simulink model "ddc_eng"  (R2012b)
(part 2 of 50)

      | pipeline_init(gcb,'latency',latency);
      settings: AttributesFormatString=Latency = %<latency>
      mask Display:
      | port_label('input', 1, 'd');
      | port_label('output', 1, 'q');
      | disp(['Z^-', num2str(latency)]);
  pipeline48 : Subsystem  AncestorBlock=casper_library_delays/pipeline  mask(pipeline){latency=2}
      mask help:
      | An explicitly laid-out delay line to avoid mapping to SRL16s
      | for use in pipelining to help achieve timing closure.
      mask init:
      | pipeline_init(gcb,'latency',latency);
      settings: AttributesFormatString=Latency = %<latency>
      mask Display:
      | port_label('input', 1, 'd');
      | port_label('output', 1, 'q');
      | disp(['Z^-', num2str(latency)]);
  pipeline49 : Subsystem  AncestorBlock=casper_library_delays/pipeline  mask(pipeline){latency=2}
      mask help:
      | An explicitly laid-out delay line to avoid mapping to SRL16s
      | for use in pipelining to help achieve timing closure.
      mask init:
      | pipeline_init(gcb,'latency',latency);
      settings: AttributesFormatString=Latency = %<latency>
      mask Display:
      | port_label('input', 1, 'd');
      | port_label('output', 1, 'q');
      | disp(['Z^-', num2str(latency)]);
  pipeline5 : Subsystem  AncestorBlock=casper_library_delays/pipeline  mask(pipeline){latency=2}
      mask help:
      | An explicitly laid-out delay line to avoid mapping to SRL16s
      | for use in pipelining to help achieve timing closure.
      mask init:
      | pipeline_init(gcb,'latency',latency);
      settings: AttributesFormatString=Latency = %<latency>
      mask Display:
      | port_label('input', 1, 'd');
      | port_label('output', 1, 'q');
      | disp(['Z^-', num2str(latency)]);
  pipeline53 : Subsystem  AncestorBlock=casper_library_delays/pipeline  mask(pipeline){latency=2}
      mask help:
      | An explicitly laid-out delay line to avoid mapping to SRL16s
      | for use in pipelining to help achieve timing closure.
      mask init:
      | pipeline_init(gcb,'latency',latency);
      settings: AttributesFormatString=Latency = %<latency>
      mask Display:
      | port_label('input', 1, 'd');
      | port_label('output', 1, 'q');
      | disp(['Z^-', num2str(latency)]);
  pipeline54 : Subsystem  AncestorBlock=casper_library_delays/pipeline  mask(pipeline){latency=2}
      mask help:
      | An explicitly laid-out delay line to avoid mapping to SRL16s
      | for use in pipelining to help achieve timing closure.
      mask init:
      | pipeline_init(gcb,'latency',latency);
      settings: AttributesFormatString=Latency = %<latency>
      mask Display:
      | port_label('input', 1, 'd');
      | port_label('output', 1, 'q');
      | disp(['Z^-', num2str(latency)]);
  pipeline55 : Subsystem  AncestorBlock=casper_library_delays/pipeline  mask(pipeline){latency=2}
      mask help:
      | An explicitly laid-out delay line to avoid mapping to SRL16s
      | for use in pipelining to help achieve timing closure.
      mask init:
      | pipeline_init(gcb,'latency',latency);
      settings: AttributesFormatString=Latency = %<latency>
      mask Display:
      | port_label('input', 1, 'd');
      | port_label('output', 1, 'q');
      | disp(['Z^-', num2str(latency)]);
  pipeline6 : Subsystem  AncestorBlock=casper_library_delays/pipeline  mask(pipeline){latency=2}
      mask help:
      | An explicitly laid-out delay line to avoid mapping to SRL16s
      | for use in pipelining to help achieve timing closure.
      mask init:
      | pipeline_init(gcb,'latency',latency);
      settings: AttributesFormatString=Latency = %<latency>
      mask Display:
      | port_label('input', 1, 'd');
      | port_label('output', 1, 'q');
      | disp(['Z^-', num2str(latency)]);
  pipeline61 : Subsystem  AncestorBlock=casper_library_delays/pipeline  mask(pipeline){latency=2}
      mask help:
      | An explicitly laid-out delay line to avoid mapping to SRL16s
      | for use in pipelining to help achieve timing closure.
      mask init:
      | pipeline_init(gcb,'latency',latency);
      settings: AttributesFormatString=Latency = %<latency>
      mask Display:
      | port_label('input', 1, 'd');
      | port_label('output', 1, 'q');
      | disp(['Z^-', num2str(latency)]);
  pipeline7 : Subsystem  AncestorBlock=casper_library_delays/pipeline  mask(pipeline){latency=2}
      mask help:
      | An explicitly laid-out delay line to avoid mapping to SRL16s
      | for use in pipelining to help achieve timing closure.
      mask init:
      | pipeline_init(gcb,'latency',latency);
      settings: AttributesFormatString=Latency = %<latency>
      mask Display:
      | port_label('input', 1, 'd');
      | port_label('output', 1, 'q');
      | disp(['Z^-', num2str(latency)]);
  pipeline8 : Subsystem  AncestorBlock=casper_library_delays/pipeline  mask(pipeline){latency=2}
      mask help:
      | An explicitly laid-out delay line to avoid mapping to SRL16s
      | for use in pipelining to help achieve timing closure.
      mask init:
      | pipeline_init(gcb,'latency',latency);
      settings: AttributesFormatString=Latency = %<latency>
      mask Display:
      | port_label('input', 1, 'd');
      | port_label('output', 1, 'q');
      | disp(['Z^-', num2str(latency)]);
  pipeline9 : Subsystem  AncestorBlock=casper_library_delays/pipeline  mask(pipeline){latency=2}
      mask help:
      | An explicitly laid-out delay line to avoid mapping to SRL16s
      | for use in pipelining to help achieve timing closure.
      mask init:
      | pipeline_init(gcb,'latency',latency);
      settings: AttributesFormatString=Latency = %<latency>
      mask Display:
      | port_label('input', 1, 'd');
      | port_label('output', 1, 'q');
      | disp(['Z^-', num2str(latency)]);
  pipeline93 : Subsystem  AncestorBlock=casper_library_delays/pipeline  mask(pipeline){latency=2}
      mask help:
      | An explicitly laid-out delay line to avoid mapping to SRL16s
      | for use in pipelining to help achieve timing closure.
      mask init:
      | pipeline_init(gcb,'latency',latency);
      settings: AttributesFormatString=Latency = %<latency>
      mask Display:
      | port_label('input', 1, 'd');
      | port_label('output', 1, 'q');
      | disp(['Z^-', num2str(latency)]);
  pipeline98 : Subsystem  AncestorBlock=casper_library_delays/pipeline  mask(pipeline){latency=2}
      mask help:
      | An explicitly laid-out delay line to avoid mapping to SRL16s
      | for use in pipelining to help achieve timing closure.
      mask init:
      | pipeline_init(gcb,'latency',latency);
      settings: AttributesFormatString=Latency = %<latency>
      mask Display:
      | port_label('input', 1, 'd');
      | port_label('output', 1, 'q');
      | disp(['Z^-', num2str(latency)]);
  pipeline99 : Subsystem  AncestorBlock=casper_library_delays/pipeline  mask(pipeline){latency=2}
      mask help:
      | An explicitly laid-out delay line to avoid mapping to SRL16s
      | for use in pipelining to help achieve timing closure.
      mask init:
      | pipeline_init(gcb,'latency',latency);
      settings: AttributesFormatString=Latency = %<latency>
      mask Display:
      | port_label('input', 1, 'd');
      | port_label('output', 1, 'q');
      | disp(['Z^-', num2str(latency)]);
  receptor_id : Subsystem  Tag=xps:sw_reg  AncestorBlock=xps_library/software register  mask(swreg){mode=fields of arbitrary size, io_dir=From Processor, io_delay=1, sample_period=1, names=[receptor_id pol0_id pol1_id], bitwidths=[14 2 2], arith_types=[0 0 0], bin_pts=[0 0 0], show_format=on}
      mask prompts: io_dir "I/O direction"; io_delay "I/O delay"; sample_period "Sample period"; names "Names [msb ... lsb]:"; bitwidths "Bitwidths [msb ... lsb]:"; arith_types "Types (ufix=0, fix=1, bool=2) [msb ... lsb]:"; bin_pts "Binary pts [msb ... lsb]:"; show_format "Print format string?"
      mask init:
      | swreg_init(gcb)
      settings: AttributesFormatString=3 inputs:uf14.0,uf2.0,uf2.0,
      mask TypeOptions mode: one value | fields of equal size | fields of arbitrary size
      mask Callback mode: swreg_cb(gcb);
      mask TypeOptions io_dir: To Processor | From Processor
      mask Callback io_dir:
      | mask_enables = get_param(gcb, 'MaskEnables');
      | mask_names = get_param(gcb, 'MaskNames');
      | if strcmp(get_param(gcb, 'io_dir'), 'To Processor'),
      |     mask_enables{ismember(mask_names, 'sample_period')} = 'off';
      | else
      |     mask_enables{ismember(mask_names, 'sample_period')} = 'on';
      | end
      | set_param(gcb, 'MaskEnables', mask_enables);
      mask Callback bitwidths:
      | blk = gcb;
      | mode = get_param(blk, 'mode');
      | current_widths = eval(get_param(blk, 'bitwidths'));
      | if (strcmp(mode, 'one value') || strcmp(mode, 'fields of equal size')) && (length(current_widths) > 1),
      |     error('Only one width may be specified for this mode.');
      | elseif strcmp(mode, 'fields of arbitrary size')
      |     current_names = textscan(strtrim(strrep(strrep(get_param(blk, 'names'), ']', ''), '[', '')), '%s');
      |     current_names = current_names{1};
      |     numios = length(current_names);
      |     if length(current_widths) ~= numios,
      |         error('%d field names specified, but %d widths?', numios, length(current_widths));
      |     end
      | end
      | total_width = 0;
      | for ctr = 1 : length(current_widths),
      |     total_width = total_width + current_widths(ctr);
      | end
      | if total_width > 32,
      |     error('Total width must be 32 or less, set to %d.', total_width);
      | end
      mask Callback arith_types:
      | blk = gcb;
      | mode = get_param(blk, 'mode');
      | current_types = eval(get_param(blk, 'arith_types'));
      | numios = length(current_types);
      | if (strcmp(mode, 'one value') || strcmp(mode, 'fields of equal size')) && (length(current_types) > 1),
      |     error('Only one type may be specified for this mode.');
      | elseif strcmp(mode, 'fields of arbitrary size')
      |     current_names = textscan(strtrim(strrep(strrep(get_param(blk, 'names'), ']', ''), '[', '')), '%s');
      |     current_names = current_names{1};
      |     numios = length(current_names);
      |     if length(current_types) ~= numios,
      |         error('%d field names specified, but %d types?', numios, length(current_types));
      |     end
      | end
      | problem = 0;
      | for ctr = 1 : numios,
      |     t = current_types(ctr);
      |     if (t < 0) || (t > 2),
      |         problem = t;
      |         ctr = numios + 1;
      |     end
      | end
      | if problem ~= 0,
      |     error('Type cannot be %i, must be 0, 1 or 2.', problem);
      | end
      mask Callback bin_pts:
      | blk = gcb;
      | mode = get_param(blk, 'mode');
      | current_bins = eval(get_param(blk, 'bin_pts'));
      | if (strcmp(mode, 'one value') || strcmp(mode, 'fields of equal size')) && (length(current_bins) > 1),
      |     error('Only one binary pt may be specified for this mode.');
      | elseif strcmp(mode, 'fields of arbitrary size')
      |     current_names = textscan(strtrim(strrep(strrep(get_param(blk, 'names'), ']', ''), '[', '')), '%s');
      |     current_names = current_names{1};
      |     numios = length(current_names);
      |     if length(current_bins) ~= numios,
      |         error('%d field names specified, but %d binary pts?', numios, length(current_bins));
      |     end
      | end
  reorder_ctrs : Subsystem  Tag=xps:sw_reg  AncestorBlock=xps_library/software register  mask(swreg){mode=fields of arbitrary size, io_dir=To Processor, io_delay=0, sample_period=1, names=[pktof0 pktof1 pktof2 pktof3], bitwidths=[8 8 8 8], arith_types=[0 0 0 0], bin_pts=[0 0 0 0], sim_port=off, show_format=on}
      mask prompts: io_dir "I/O direction"; io_delay "I/O delay"; sample_period "Sample period"; names "Names [msb ... lsb]:"; bitwidths "Bitwidths [msb ... lsb]:"; arith_types "Types (ufix=0, fix=1, bool=2) [msb ... lsb]:"; bin_pts "Binary pts [msb ... lsb]:"; sim_port "Provide sim input/output?"; show_format "Print format string?"
      mask init:
      | swreg_init(gcb)
      settings: AttributesFormatString=4 outputs:uf8.0,uf8.0,uf8.0,uf8.0,
      mask TypeOptions mode: one value | fields of equal size | fields of arbitrary size
      mask Callback mode: swreg_cb(gcb);
      mask TypeOptions io_dir: To Processor | From Processor
      mask Callback io_dir:
      | mask_enables = get_param(gcb, 'MaskEnables');
      | mask_names = get_param(gcb, 'MaskNames');
      | if strcmp(get_param(gcb, 'io_dir'), 'To Processor'),
      |     mask_enables{ismember(mask_names, 'sample_period')} = 'off';
      | else
      |     mask_enables{ismember(mask_names, 'sample_period')} = 'on';
      | end
      | set_param(gcb, 'MaskEnables', mask_enables);
      mask Callback bitwidths:
      | blk = gcb;
      | mode = get_param(blk, 'mode');
      | current_widths = eval(get_param(blk, 'bitwidths'));
      | if (strcmp(mode, 'one value') || strcmp(mode, 'fields of equal size')) && (length(current_widths) > 1),
      |     error('Only one width may be specified for this mode.');
      | elseif strcmp(mode, 'fields of arbitrary size')
      |     current_names = textscan(strtrim(strrep(strrep(get_param(blk, 'names'), ']', ''), '[', '')), '%s');
      |     current_names = current_names{1};
      |     numios = length(current_names);
      |     if length(current_widths) ~= numios,
      |         error('%d field names specified, but %d widths?', numios, length(current_widths));
      |     end
      | end
      | total_width = 0;
      | for ctr = 1 : length(current_widths),
      |     total_width = total_width + current_widths(ctr);
      | end
      | if total_width > 32,
      |     error('Total width must be 32 or less, set to %d.', total_width);
      | end
      mask Callback arith_types:
      | blk = gcb;
      | mode = get_param(blk, 'mode');
      | current_types = eval(get_param(blk, 'arith_types'));
      | numios = length(current_types);
      | if (strcmp(mode, 'one value') || strcmp(mode, 'fields of equal size')) && (length(current_types) > 1),
      |     error('Only one type may be specified for this mode.');
      | elseif strcmp(mode, 'fields of arbitrary size')
      |     current_names = textscan(strtrim(strrep(strrep(get_param(blk, 'names'), ']', ''), '[', '')), '%s');
      |     current_names = current_names{1};
      |     numios = length(current_names);
      |     if length(current_types) ~= numios,
      |         error('%d field names specified, but %d types?', numios, length(current_types));
      |     end
      | end
      | problem = 0;
      | for ctr = 1 : numios,
      |     t = current_types(ctr);
      |     if (t < 0) || (t > 2),
      |         problem = t;
      |         ctr = numios + 1;
      |     end
      | end
      | if problem ~= 0,
      |     error('Type cannot be %i, must be 0, 1 or 2.', problem);
      | end
      mask Callback bin_pts:
      | blk = gcb;
      | mode = get_param(blk, 'mode');
      | current_bins = eval(get_param(blk, 'bin_pts'));
      | if (strcmp(mode, 'one value') || strcmp(mode, 'fields of equal size')) && (length(current_bins) > 1),
      |     error('Only one binary pt may be specified for this mode.');
      | elseif strcmp(mode, 'fields of arbitrary size')
      |     current_names = textscan(strtrim(strrep(strrep(get_param(blk, 'names'), ']', ''), '[', '')), '%s');
      |     current_names = current_names{1};
      |     numios = length(current_names);
      |     if length(current_bins) ~= numios,
      |         error('%d field names specified, but %d binary pts?', numios, length(current_bins));
      |     end
      | end
  reorder_ctrs1 : Subsystem  Tag=xps:sw_reg  AncestorBlock=xps_library/software register  mask(swreg){mode=fields of arbitrary size, io_dir=To Processor, io_delay=0, sample_period=1, names=[discard timestep_error mcnt_relock recverr0 recverr1], bitwidths=[6 6 6 6 6], arith_types=[0 0 0 0 0], bin_pts=[0 0 0 0 0], sim_port=off, show_format=on}
      mask prompts: io_dir "I/O direction"; io_delay "I/O delay"; sample_period "Sample period"; names "Names [msb ... lsb]:"; bitwidths "Bitwidths [msb ... lsb]:"; arith_types "Types (ufix=0, fix=1, bool=2) [msb ... lsb]:"; bin_pts "Binary pts [msb ... lsb]:"; sim_port "Provide sim input/output?"; show_format "Print format string?"
      mask init:
      | swreg_init(gcb)
      settings: AttributesFormatString=5 outputs:uf6.0,uf6.0,uf6.0,uf6.0,uf6.0,
      mask TypeOptions mode: one value | fields of equal size | fields of arbitrary size
      mask Callback mode: swreg_cb(gcb);
      mask TypeOptions io_dir: To Processor | From Processor
      mask Callback io_dir:
      | mask_enables = get_param(gcb, 'MaskEnables');
      | mask_names = get_param(gcb, 'MaskNames');
      | if strcmp(get_param(gcb, 'io_dir'), 'To Processor'),
      |     mask_enables{ismember(mask_names, 'sample_period')} = 'off';
      | else
      |     mask_enables{ismember(mask_names, 'sample_period')} = 'on';
      | end
      | set_param(gcb, 'MaskEnables', mask_enables);
      mask Callback bitwidths:
      | blk = gcb;
      | mode = get_param(blk, 'mode');
      | current_widths = eval(get_param(blk, 'bitwidths'));
      | if (strcmp(mode, 'one value') || strcmp(mode, 'fields of equal size')) && (length(current_widths) > 1),
      |     error('Only one width may be specified for this mode.');
      | elseif strcmp(mode, 'fields of arbitrary size')
      |     current_names = textscan(strtrim(strrep(strrep(get_param(blk, 'names'), ']', ''), '[', '')), '%s');
      |     current_names = current_names{1};
      |     numios = length(current_names);
      |     if length(current_widths) ~= numios,
      |         error('%d field names specified, but %d widths?', numios, length(current_widths));
      |     end
      | end
      | total_width = 0;
      | for ctr = 1 : length(current_widths),
      |     total_width = total_width + current_widths(ctr);
      | end
      | if total_width > 32,
      |     error('Total width must be 32 or less, set to %d.', total_width);
      | end
      mask Callback arith_types:
      | blk = gcb;
      | mode = get_param(blk, 'mode');
      | current_types = eval(get_param(blk, 'arith_types'));
      | numios = length(current_types);
      | if (strcmp(mode, 'one value') || strcmp(mode, 'fields of equal size')) && (length(current_types) > 1),
      |     error('Only one type may be specified for this mode.');
      | elseif strcmp(mode, 'fields of arbitrary size')
      |     current_names = textscan(strtrim(strrep(strrep(get_param(blk, 'names'), ']', ''), '[', '')), '%s');
      |     current_names = current_names{1};
      |     numios = length(current_names);
      |     if length(current_types) ~= numios,
      |         error('%d field names specified, but %d types?', numios, length(current_types));
      |     end
      | end
      | problem = 0;
      | for ctr = 1 : numios,
      |     t = current_types(ctr);
      |     if (t < 0) || (t > 2),
      |         problem = t;
      |         ctr = numios + 1;
      |     end
      | end
      | if problem ~= 0,
      |     error('Type cannot be %i, must be 0, 1 or 2.', problem);
      | end
      mask Callback bin_pts:
      | blk = gcb;
      | mode = get_param(blk, 'mode');
      | current_bins = eval(get_param(blk, 'bin_pts'));
      | if (strcmp(mode, 'one value') || strcmp(mode, 'fields of equal size')) && (length(current_bins) > 1),
      |     error('Only one binary pt may be specified for this mode.');
      | elseif strcmp(mode, 'fields of arbitrary size')
      |     current_names = textscan(strtrim(strrep(strrep(get_param(blk, 'names'), ']', ''), '[', '')), '%s');
      |     current_names = current_names{1};
      |     numios = length(current_names);
      |     if length(current_bins) ~= numios,
      |         error('%d field names specified, but %d binary pts?', numios, length(current_bins));
      |     end
      | end
  spead_ctrs : Subsystem  Tag=xps:sw_reg  AncestorBlock=xps_library/software register  mask(swreg){mode=fields of equal size, io_dir=To Processor, io_delay=0, sample_period=1, names=[rx_cnt0 rx_cnt1 rx_cnt2 rx_cnt3 err_cnt0 err_cnt1 err_cnt2 err_cnt3], bitwidths=4, arith_types=0, bin_pts=0, sim_port=off, show_format=on}
      mask prompts: io_dir "I/O direction"; io_delay "I/O delay"; sample_period "Sample period"; names "Names [msb ... lsb]:"; bitwidths "Bitwidth:"; arith_types "Type (ufix=0, fix=1, bool=2):"; bin_pts "Binary pt:"; sim_port "Provide sim input/output?"; show_format "Print format string?"
      mask init:
      | swreg_init(gcb)
      settings: AttributesFormatString=8 outputs:uf4.0,uf4.0,uf4.0,uf4.0,uf4.0,uf4.0,uf4.0,uf4.0,
      mask TypeOptions mode: one value | fields of equal size | fields of arbitrary size
      mask Callback mode: swreg_cb(gcb);
      mask TypeOptions io_dir: To Processor | From Processor
      mask Callback io_dir:
      | mask_enables = get_param(gcb, 'MaskEnables');
      | mask_names = get_param(gcb, 'MaskNames');
      | if strcmp(get_param(gcb, 'io_dir'), 'To Processor'),
      |     mask_enables{ismember(mask_names, 'sample_period')} = 'off';
      | else
      |     mask_enables{ismember(mask_names, 'sample_period')} = 'on';
      | end
      | set_param(gcb, 'MaskEnables', mask_enables);
      mask Callback bitwidths:
      | blk = gcb;
      | mode = get_param(blk, 'mode');
      | current_widths = eval(get_param(blk, 'bitwidths'));
      | if (strcmp(mode, 'one value') || strcmp(mode, 'fields of equal size')) && (length(current_widths) > 1),
      |     error('Only one width may be specified for this mode.');
      | elseif strcmp(mode, 'fields of arbitrary size')
      |     current_names = textscan(strtrim(strrep(strrep(get_param(blk, 'names'), ']', ''), '[', '')), '%s');
      |     current_names = current_names{1};
      |     numios = length(current_names);
      |     if length(current_widths) ~= numios,
      |         error('%d field names specified, but %d widths?', numios, length(current_widths));
      |     end
      | end
      | total_width = 0;
      | for ctr = 1 : length(current_widths),
      |     total_width = total_width + current_widths(ctr);
      | end
      | if total_width > 32,
      |     error('Total width must be 32 or less, set to %d.', total_width);
      | end
      mask Callback arith_types:
      | blk = gcb;
      | mode = get_param(blk, 'mode');
      | current_types = eval(get_param(blk, 'arith_types'));
      | numios = length(current_types);
      | if (strcmp(mode, 'one value') || strcmp(mode, 'fields of equal size')) && (length(current_types) > 1),
      |     error('Only one type may be specified for this mode.');
      | elseif strcmp(mode, 'fields of arbitrary size')
      |     current_names = textscan(strtrim(strrep(strrep(get_param(blk, 'names'), ']', ''), '[', '')), '%s');
      |     current_names = current_names{1};
      |     numios = length(current_names);
      |     if length(current_types) ~= numios,
      |         error('%d field names specified, but %d types?', numios, length(current_types));
      |     end
      | end
      | problem = 0;
      | for ctr = 1 : numios,
      |     t = current_types(ctr);
      |     if (t < 0) || (t > 2),
      |         problem = t;
      |         ctr = numios + 1;
      |     end
      | end
      | if problem ~= 0,
      |     error('Type cannot be %i, must be 0, 1 or 2.', problem);
      | end
      mask Callback bin_pts:
      | blk = gcb;
      | mode = get_param(blk, 'mode');
      | current_bins = eval(get_param(blk, 'bin_pts'));
      | if (strcmp(mode, 'one value') || strcmp(mode, 'fields of equal size')) && (length(current_bins) > 1),
      |     error('Only one binary pt may be specified for this mode.');
      | elseif strcmp(mode, 'fields of arbitrary size')
      |     current_names = textscan(strtrim(strrep(strrep(get_param(blk, 'names'), ']', ''), '[', '')), '%s');
      |     current_names = current_names{1};
      |     numios = length(current_names);
      |     if length(current_bins) ~= numios,
      |         error('%d field names specified, but %d binary pts?', numios, length(current_bins));
      |     end
      | end
  spead_of_ctr : Subsystem  Tag=xps:sw_reg  AncestorBlock=xps_library/software register  mask(swreg){mode=fields of equal size, io_dir=To Processor, io_delay=0, sample_period=1, names=[pol0 pol1], bitwidths=16, arith_types=0, bin_pts=0, sim_port=off, show_format=on}
      mask prompts: io_dir "I/O direction"; io_delay "I/O delay"; sample_period "Sample period"; names "Names [msb ... lsb]:"; bitwidths "Bitwidth:"; arith_types "Type (ufix=0, fix=1, bool=2):"; bin_pts "Binary pt:"; sim_port "Provide sim input/output?"; show_format "Print format string?"
      mask init:
      | swreg_init(gcb)
      settings: AttributesFormatString=2 outputs:uf16.0,uf16.0,
      mask TypeOptions mode: one value | fields of equal size | fields of arbitrary size
      mask Callback mode: swreg_cb(gcb);
      mask TypeOptions io_dir: To Processor | From Processor
      mask Callback io_dir:
      | mask_enables = get_param(gcb, 'MaskEnables');
      | mask_names = get_param(gcb, 'MaskNames');
      | if strcmp(get_param(gcb, 'io_dir'), 'To Processor'),
      |     mask_enables{ismember(mask_names, 'sample_period')} = 'off';
      | else
      |     mask_enables{ismember(mask_names, 'sample_period')} = 'on';
      | end
      | set_param(gcb, 'MaskEnables', mask_enables);
      mask Callback bitwidths:
      | blk = gcb;
      | mode = get_param(blk, 'mode');
      | current_widths = eval(get_param(blk, 'bitwidths'));
      | if (strcmp(mode, 'one value') || strcmp(mode, 'fields of equal size')) && (length(current_widths) > 1),
      |     error('Only one width may be specified for this mode.');
      | elseif strcmp(mode, 'fields of arbitrary size')
      |     current_names = textscan(strtrim(strrep(strrep(get_param(blk, 'names'), ']', ''), '[', '')), '%s');
      |     current_names = current_names{1};
      |     numios = length(current_names);
      |     if length(current_widths) ~= numios,
      |         error('%d field names specified, but %d widths?', numios, length(current_widths));
      |     end
      | end
      | total_width = 0;
      | for ctr = 1 : length(current_widths),
      |     total_width = total_width + current_widths(ctr);
      | end
      | if total_width > 32,
      |     error('Total width must be 32 or less, set to %d.', total_width);
      | end
      mask Callback arith_types:
      | blk = gcb;
      | mode = get_param(blk, 'mode');
      | current_types = eval(get_param(blk, 'arith_types'));
      | numios = length(current_types);
      | if (strcmp(mode, 'one value') || strcmp(mode, 'fields of equal size')) && (length(current_types) > 1),
      |     error('Only one type may be specified for this mode.');
      | elseif strcmp(mode, 'fields of arbitrary size')
      |     current_names = textscan(strtrim(strrep(strrep(get_param(blk, 'names'), ']', ''), '[', '')), '%s');
      |     current_names = current_names{1};
      |     numios = length(current_names);
      |     if length(current_types) ~= numios,
      |         error('%d field names specified, but %d types?', numios, length(current_types));
      |     end
      | end
      | problem = 0;
      | for ctr = 1 : numios,
      |     t = current_types(ctr);
      |     if (t < 0) || (t > 2),
      |         problem = t;
      |         ctr = numios + 1;
      |     end
      | end
      | if problem ~= 0,
      |     error('Type cannot be %i, must be 0, 1 or 2.', problem);
      | end
      mask Callback bin_pts:
      | blk = gcb;
      | mode = get_param(blk, 'mode');
      | current_bins = eval(get_param(blk, 'bin_pts'));
      | if (strcmp(mode, 'one value') || strcmp(mode, 'fields of equal size')) && (length(current_bins) > 1),
      |     error('Only one binary pt may be specified for this mode.');
      | elseif strcmp(mode, 'fields of arbitrary size')
      |     current_names = textscan(strtrim(strrep(strrep(get_param(blk, 'names'), ']', ''), '[', '')), '%s');
      |     current_names = current_names{1};
      |     numios = length(current_names);
      |     if length(current_bins) ~= numios,
      |         error('%d field names specified, but %d binary pts?', numios, length(current_bins));
      |     end
      | end
  spead_pack0 : Subsystem  Tag=casper:spead_pack  AncestorBlock=casper_library_communications/spead_pack  mask(pkt_pack_mask){max_pkt_len_bits=10, header_ids=0x1600, 0x3101, 0x3102, header_ind_ids=0x3300, spead_msw=64, spead_lsw=48, spead_version=4, bytes_per_word=8}
      mask prompts: max_pkt_len_bits "Max pkt length, 2^? 64-bit words"; header_ids "SPEAD direct address IDs (decimal)"; header_ind_ids "SPEAD indirect address IDs (decimal)"; spead_msw "SPEAD Flavour (MSw)"; spead_lsw "SPEAD Flavour (LSw)"; spead_version "SPEAD version"; bytes_per_word "Word size, in bytes"
      mask help:
      | This block generates SPEAD-compliant packets from a datastream.
      |
      | Packets are created with a fixed header followed by a number of 64-bit items.
      |
      | Requires a 64-bit data stream.
      |
      | The data_ready signal is one cycle BEFORE valid data! Does not have to be with a valid signal either.
      mask init:
      | if floor(log2(bytes_per_word)) ~= log2(bytes_per_word)
      |     error('Bytes per word should be a power of two.');
      | end
      | 
      | spead_pack_init(gcb)
  spead_pack1 : Subsystem  Tag=casper:spead_pack  AncestorBlock=casper_library_communications/spead_pack  mask(pkt_pack_mask){max_pkt_len_bits=10, header_ids=0x1600, 0x3101, 0x3102, header_ind_ids=0x3300, spead_msw=64, spead_lsw=48, spead_version=4, bytes_per_word=8}
      mask prompts: max_pkt_len_bits "Max pkt length, 2^? 64-bit words"; header_ids "SPEAD direct address IDs (decimal)"; header_ind_ids "SPEAD indirect address IDs (decimal)"; spead_msw "SPEAD Flavour (MSw)"; spead_lsw "SPEAD Flavour (LSw)"; spead_version "SPEAD version"; bytes_per_word "Word size, in bytes"
      mask help:
      | This block generates SPEAD-compliant packets from a datastream.
      |
      | Packets are created with a fixed header followed by a number of 64-bit items.
      |
      | Requires a 64-bit data stream.
      |
      | The data_ready signal is one cycle BEFORE valid data! Does not have to be with a valid signal either.
      mask init:
      | if floor(log2(bytes_per_word)) ~= log2(bytes_per_word)
      |     error('Bytes per word should be a power of two.');
      | end
      | 
      | spead_pack_init(gcb)
  status : Subsystem  Tag=xps:sw_reg  AncestorBlock=xps_library/software register  mask(swreg){mode=fields of arbitrary size, io_dir=To Processor, io_delay=0, sample_period=1, names=[gbe0_linkup gbe1_linkup gbe2_linkup gbe3_linkup], bitwidths=[1 1 1 1], arith_types=[2 2 2 2], bin_pts=[0 0 0 0], sim_port=off, show_format=on}
      mask prompts: io_dir "I/O direction"; io_delay "I/O delay"; sample_period "Sample period"; names "Names [msb ... lsb]:"; bitwidths "Bitwidths [msb ... lsb]:"; arith_types "Types (ufix=0, fix=1, bool=2) [msb ... lsb]:"; bin_pts "Binary pts [msb ... lsb]:"; sim_port "Provide sim input/output?"; show_format "Print format string?"
      mask init:
      | swreg_init(gcb)
      settings: AttributesFormatString=4 outputs:b,b,b,b,
      mask TypeOptions mode: one value | fields of equal size | fields of arbitrary size
      mask Callback mode: swreg_cb(gcb);
      mask TypeOptions io_dir: To Processor | From Processor
      mask Callback io_dir:
      | mask_enables = get_param(gcb, 'MaskEnables');
      | mask_names = get_param(gcb, 'MaskNames');
      | if strcmp(get_param(gcb, 'io_dir'), 'To Processor'),
      |     mask_enables{ismember(mask_names, 'sample_period')} = 'off';
      | else
      |     mask_enables{ismember(mask_names, 'sample_period')} = 'on';
      | end
      | set_param(gcb, 'MaskEnables', mask_enables);
      mask Callback bitwidths:
      | blk = gcb;
      | mode = get_param(blk, 'mode');
      | current_widths = eval(get_param(blk, 'bitwidths'));
      | if (strcmp(mode, 'one value') || strcmp(mode, 'fields of equal size')) && (length(current_widths) > 1),
      |     error('Only one width may be specified for this mode.');
      | elseif strcmp(mode, 'fields of arbitrary size')
      |     current_names = textscan(strtrim(strrep(strrep(get_param(blk, 'names'), ']', ''), '[', '')), '%s');
      |     current_names = current_names{1};
      |     numios = length(current_names);
      |     if length(current_widths) ~= numios,
      |         error('%d field names specified, but %d widths?', numios, length(current_widths));
      |     end
      | end
      | total_width = 0;
      | for ctr = 1 : length(current_widths),
      |     total_width = total_width + current_widths(ctr);
      | end
      | if total_width > 32,
      |     error('Total width must be 32 or less, set to %d.', total_width);
      | end
      mask Callback arith_types:
      | blk = gcb;
      | mode = get_param(blk, 'mode');
      | current_types = eval(get_param(blk, 'arith_types'));
      | numios = length(current_types);
      | if (strcmp(mode, 'one value') || strcmp(mode, 'fields of equal size')) && (length(current_types) > 1),
      |     error('Only one type may be specified for this mode.');
      | elseif strcmp(mode, 'fields of arbitrary size')
      |     current_names = textscan(strtrim(strrep(strrep(get_param(blk, 'names'), ']', ''), '[', '')), '%s');
      |     current_names = current_names{1};
      |     numios = length(current_names);
      |     if length(current_types) ~= numios,
      |         error('%d field names specified, but %d types?', numios, length(current_types));
      |     end
      | end
      | problem = 0;
      | for ctr = 1 : numios,
      |     t = current_types(ctr);
      |     if (t < 0) || (t > 2),
      |         problem = t;
      |         ctr = numios + 1;
      |     end
      | end
      | if problem ~= 0,
      |     error('Type cannot be %i, must be 0, 1 or 2.', problem);
      | end
      mask Callback bin_pts:
      | blk = gcb;
      | mode = get_param(blk, 'mode');
      | current_bins = eval(get_param(blk, 'bin_pts'));
      | if (strcmp(mode, 'one value') || strcmp(mode, 'fields of equal size')) && (length(current_bins) > 1),
      |     error('Only one binary pt may be specified for this mode.');
      | elseif strcmp(mode, 'fields of arbitrary size')
      |     current_names = textscan(strtrim(strrep(strrep(get_param(blk, 'names'), ']', ''), '[', '')), '%s');
      |     current_names = current_names{1};
      |     numios = length(current_names);
      |     if length(current_bins) ~= numios,
      |         error('%d field names specified, but %d binary pts?', numios, length(current_bins));
      |     end
      | end
  sync_gen : Subsystem  mask{zerolsbs=((15 + 1) + 8)}
      mask prompts: zerolsbs "No. LSBs to be zero:"
  tvg_flags : Subsystem  Tag=xps:sw_reg  AncestorBlock=xps_library/software register  mask(swreg){mode=fields of arbitrary size, io_dir=From Processor, io_delay=1, sample_period=1, names=[pfb_of timestep_error missing mcnt_relock discarded pktof fifo_of spead_error adc_or0 adc_or1 ndiode0 ndiode1], bitwidths=[2 1 1 1 1 1 1 1 1 1 1 1], arith_types=[0 0 0 0 0 0 0 0 0 0 0 0], bin_pts=[0 0 0 0 0 0 0 0 0 0 0 0], sim_port=off, show_format=off}
      mask prompts: io_dir "I/O direction"; io_delay "I/O delay"; sample_period "Sample period"; names "Names [msb ... lsb]:"; bitwidths "Bitwidths [msb ... lsb]:"; arith_types "Types (ufix=0, fix=1, bool=2) [msb ... lsb]:"; bin_pts "Binary pts [msb ... lsb]:"; sim_port "Provide sim input/output?"; show_format "Print format string?"
      mask init:
      | swreg_init(gcb)
      settings: AttributesFormatString=12 inputs
      mask TypeOptions mode: one value | fields of equal size | fields of arbitrary size
      mask Callback mode: swreg_cb(gcb);
      mask TypeOptions io_dir: To Processor | From Processor
      mask Callback io_dir:
      | mask_enables = get_param(gcb, 'MaskEnables');
      | mask_names = get_param(gcb, 'MaskNames');
      | if strcmp(get_param(gcb, 'io_dir'), 'To Processor'),
      |     mask_enables{ismember(mask_names, 'sample_period')} = 'off';
      | else
      |     mask_enables{ismember(mask_names, 'sample_period')} = 'on';
      | end
      | set_param(gcb, 'MaskEnables', mask_enables);
      mask Callback bitwidths:
      | swreg_maskcheck(gcb);
      | % blk = gcb;
      | % mode = get_param(blk, 'mode');
      | % current_widths = eval(get_param(blk, 'bitwidths'));
      | % if (strcmp(mode, 'one value') || strcmp(mode, 'fields of equal size')) && (length(current_widths) > 1),
      | %     error('Only one width may be specified for this mode.');
      | % elseif strcmp(mode, 'fields of arbitrary size')
      | %     current_names = textscan(strtrim(strrep(strrep(get_param(blk, 'names'), ']', ''), '[', '')), '%s');
      | %     current_names = current_names{1};
      | %     numios = length(current_names);
      | %     if length(current_widths) ~= numios,
      | %         error('%d field names specified, but %d widths?', numios, length(current_widths));
      | %     end
      | % end
      | % total_width = 0;
      | % for ctr = 1 : length(current_widths),
      | %     total_width = total_width + current_widths(ctr);
      | % end
      | % if total_width > 32,
      | %     error('Total width must be 32 or less, set to %d.', total_width);
      | % end
      mask Callback arith_types:
      | [numios, ~, ~, ~, current_types] = swreg_maskcheck(gcb);
      | % blk = gcb;
      | % mode = get_param(blk, 'mode');
      | % current_types = eval(get_param(blk, 'arith_types'));
      | % numios = length(current_types);
      | % if (strcmp(mode, 'one value') || strcmp(mode, 'fields of equal size')) && (length(current_types) > 1),
      | %     error('Only one type may be specified for this mode.');
      | % elseif strcmp(mode, 'fields of arbitrary size')
      | %     current_names = textscan(strtrim(strrep(strrep(get_param(blk, 'names'), ']', ''), '[', '')), '%s');
      | %     current_names = current_names{1};
      | %     numios = length(current_names);
      | %     if length(current_types) ~= numios,
      | %         error('%d field names specified, but %d types?', numios, length(current_types));
      | %     end
      | % end
      | problem = 0;
      | for ctr = 1 : numios,
      |     t = current_types(ctr);
      |     if (t < 0) || (t > 2),
      |         problem = t;
      |         ctr = numios + 1;
      |     end
      | end
      | if problem ~= 0,
      |     error('Type cannot be %i, must be 0, 1 or 2.', problem);
      | end
      mask Callback bin_pts:
      | swreg_maskcheck(gcb);
      | % blk = gcb;
      | % mode = get_param(blk, 'mode');
      | % current_bins = eval(get_param(blk, 'bin_pts'));
      | % if (strcmp(mode, 'one value') || strcmp(mode, 'fields of equal size')) && (length(current_bins) > 1),
      | %     error('Only one binary pt may be specified for this mode.');
      | % elseif strcmp(mode, 'fields of arbitrary size')
      | %     current_names = textscan(strtrim(strrep(strrep(get_param(blk, 'names'), ']', ''), '[', '')), '%s');
      | %     current_names = current_names{1};
      | %     numios = length(current_names);
      | %     if length(current_bins) ~= numios,
      | %         error('%d field names specified, but %d binary pts?', numios, length(current_bins));
      | %     end
      | % end
  unpack_and_reorder : Subsystem  mask{n_bits_packet_size=9, n_bits_timestep=9+3, n_bits_fifo_depth=4, n_bits_buffer_depth=4, bram_latency=1}
      mask prompts: n_bits_packet_size "Packet size (2^? 80-bit words after unpacking)"; n_bits_timestep "Packet timestep (2^?)"; n_bits_fifo_depth "FIFO depth (2^? packets)"; n_bits_buffer_depth "Reorder buffer size (2^? packets)"; bram_latency "BRAM latency"
  xps : xps_library/XSG core config  Tag=xps:xsg  hw_sys=ROACH2:sx475t  clk_src=sys_clk  ROACH_clk_src=adc0_clk  ROACH2_clk_src=sys_clk  MKDIG_clk_src=sys_clk  clk_rate=228  sample_period=1  synthesis_tool=XST
  tag scope: cnt_rst=global, s64_d0=global, s64_d1=global, s64_d2=global, s64_d3=global, s64_eof0=global, s64_eof1=global, s64_eof2=global, s64_eof3=global, s64_v0=global, s64_v1=global, s64_v2=global, s64_v3=global, spead_d0=global, spead_d1=global, spead_dv0=global, spead_dv1=global, spead_eof0=global, spead_eof1=global, spead_of0=global, spead_of1=global, tvg_pfb_flags_en=global, tvg_unpack_flags_en=global
  wires:
  [sync80] -> pipeline1/1(d)
  [valid80] -> pipeline17/1(d)
  bus_expand3/1(msb_out8) -> dec_fir_async/3(real1)
  bus_expand3/2(out7) -> dec_fir_async/5(real2)
  bus_expand3/3(out6) -> dec_fir_async/7(real3)
  bus_expand3/4(out5) -> dec_fir_async/9(real4)
  bus_expand3/5(out4) -> dec_fir_async/11(real5)
  bus_expand3/6(out3) -> dec_fir_async/13(real6)
  bus_expand3/7(out2) -> dec_fir_async/15(real7)
  bus_expand3/8(lsb_out1) -> dec_fir_async/17(real8)
  bus_expand4/8(lsb_out1) -> dec_fir_async/18(imag8)
  bus_expand4/7(out2) -> dec_fir_async/16(imag7)
  bus_expand4/6(out3) -> dec_fir_async/14(imag6)
  bus_expand4/5(out4) -> dec_fir_async/12(imag5)
  bus_expand4/4(out5) -> dec_fir_async/10(imag4)
  bus_expand4/3(out6) -> dec_fir_async/8(imag3)
  bus_expand4/2(out7) -> dec_fir_async/6(imag2)
  bus_expand4/1(msb_out8) -> dec_fir_async/4(imag1)
  [d80_adc0] -> pipeline20/1(d)
  [d80_adc1] -> pipeline21/1(d)
  dec_fir_async/1(sync_out) -> [sync_filt]
  dec_fir_async/2(dout) -> bus_expand7/1(bus_in), bus_expand5/1(bus_in)
  bus_expand5/2(lsb_out1) -> [d10_filt_1]
  dec_fir_async/3(dv_out) -> filtout/3(we), [dv_filt]
  pipeline1/1(q) -> dec_fir_async/1(sync_in)
  pipeline17/1(q) -> dec_fir_async/2(dv_in)
  pipeline20/1(q) -> bus_expand3/1(bus_in)
  pipeline21/1(q) -> bus_expand4/1(bus_in)
  [hdr_0x3101] -> bus_create9/1(in1)
  [pol0_id] -> bus_create9/2(in2)
  [hdr_0x3101] -> bus_create1/1(in1)
  [pol1_id] -> bus_create1/2(in2)
  [pkt_time48] -> spead_pack0/4(hdr_heap_id), spead_pack0/8(hdr5_0x1600_DIR)  "timein0"
  bus_create9/1(bus_out) -> spead_pack0/9(hdr6_0x3101_DIR)
  [status0] -> spead_pack0/10(hdr7_0x3102_DIR)
  bus_create1/1(bus_out) -> spead_pack1/9(hdr6_0x3101_DIR)
  [status1] -> spead_pack1/10(hdr7_0x3102_DIR)
  [pkt_start] -> spead_pack0/1(data64_ready)  "r64_00"
  [pkt_dv] -> spead_pack0/2(data64_valid)  "v64_00"
  [pkt_d64_0] -> spead_pack0/3(data64)  "d64_00"
  [spead_heapsize] -> spead_pack0/5(hdr_heap_size)
  [spead_heapoffset] -> spead_pack0/6(hdr_heap_offset)
  [spead_pktlen] -> spead_pack0/7(hdr_pkt_len_words)
  [spead_heapsize] -> spead_pack1/5(hdr_heap_size)
  [spead_heapoffset] -> spead_pack1/6(hdr_heap_offset)
  [spead_pktlen] -> spead_pack1/7(hdr_pkt_len_words)
  spead_pack1/4(data_overflow) -> counter4/2, [spead_of1]
  [adc_data_offset] -> spead_pack0/11(hdr8_0x3300)
  [adc_data_offset] -> spead_pack1/11(hdr8_0x3300)
  Constant26/1 -> [spead_heapsize]
  Constant27/1 -> [spead_pktlen]
  Constant45/1 -> [spead_heapoffset]
  spead_pack0/4(data_overflow) -> counter3/2, [spead_of0]
  spead_pack0/3(eof) -> [spead_eof0]
  spead_pack0/1(data_out) -> [spead_d0]  "packd"
  spead_pack0/2(valid_out) -> [spead_dv0]  "packv"
  spead_pack1/1(data_out) -> [spead_d1]
  spead_pack1/2(valid_out) -> [spead_dv1]
  spead_pack1/3(eof) -> [spead_eof1]
  Constant8/1 -> [adc_data_offset]
  [time80_48] -> pipeline23/1(d)
  pipeline23/1(q) -> [time48_filt]
  [time48_filt] -> Register3/1
  gbe_porttx/1(in_reg) -> [s64_port]
  gbe_iptx0/1(in_reg) -> [s64_ip0]
  gbe_iptx1/1(in_reg) -> [s64_ip1]
  Constant9/1 -> gbe_porttx/1(sim_1)
  Constant10/1 -> gbe_iptx0/1(sim_1)
  Constant12/1 -> gbe_iptx1/1(sim_1)
  Constant15/1 -> digitiser_id/1(sim_1)
  Constant17/1 -> receptor_id/1(sim_1)
  bus_create/1(bus_out) -> [hdr_0x3101]
  Constant16/1 -> digitiser_id/2(sim_2)
  receptor_id/1(in_receptor_id) -> bus_create/3(in3)
  receptor_id/2(in_pol0_id) -> [pol0_id]
  receptor_id/3(in_pol1_id) -> [pol1_id]
  Constant6/1 -> receptor_id/2(sim_2)
  Constant19/1 -> receptor_id/3(sim_3)
  digitiser_id/1(in_digitiser_serial) -> bus_create/1(in1)
  digitiser_id/2(in_digitiser_type) -> bus_create/2(in2)
  Constant1/1 -> [status3], [status2], [status1], [status0]  "status"
  [sync_filt] -> 10_to_64_new/1(sync_in)
  [dv_filt] -> 10_to_64_new/2(dv_in), Register3/2
  [d10_filt_0] -> 10_to_64_new/3(pol0_10)
  [d10_filt_1] -> 10_to_64_new/4(pol1_10)
  10_to_64_new/5(pkt_start) -> Register2/2, gap_enforcer/1(pkt_start)
  10_to_64_new/1(sync_out) -> Terminator3/1
  10_to_64_new/2(dv_out) -> gap_enforcer/2(en)
  10_to_64_new/3(d64_out0) -> Concat1/1
  10_to_64_new/4(d64_out1) -> Concat1/2
  Concat1/1 -> gap_enforcer/3(din)
  Register3/1 -> Register2/1
  Register2/1 -> Register7/1
  gap_enforcer/1(pkt_start_out) -> Register7/2, Logical8/1, [pkt_start]
  [cnt_rst] -> pipeline24/1(d)
  pipeline24/1(q) -> counter2/1
  gap_enforcer/4(full) -> counter2/2
  counter2/1 -> gap_enf_full/1(out_reg)
  gap_enforcer/3(dout) -> bus_expand8/1(bus_in)
  gap_enforcer/2(dvalid) -> packed_p1/2(we), packed_p0/2(we), [pkt_dv]
  bus_expand8/1(msb_out2) -> packed_p0/1(in_p0), [pkt_d64_0]
  bus_expand8/2(lsb_out1) -> packed_p1/1(in_p0), [pkt_d64_1]
  Register7/1 -> Slice1/1
  [pkt_start] -> spead_pack1/1(data64_ready)
  [pkt_dv] -> spead_pack1/2(data64_valid)
  [pkt_d64_1] -> spead_pack1/3(data64)
  [pkt_time48] -> spead_pack1/4(hdr_heap_id), spead_pack1/8(hdr5_0x1600_DIR)
  [cnt_rst] -> pipeline25/1(d)
  pipeline25/1(q) -> counter4/1, counter3/1
  counter3/1 -> spead_of_ctr/1(out_pol0)
  counter4/1 -> spead_of_ctr/2(out_pol1)
  bus_create2/1(bus_out) -> [pkt_time48]
  Slice1/1 -> bus_create2/2(in2)
  Constant/1 -> bus_create2/1(in1)
  bus_expand5/1(msb_out2) -> [d10_filt_0]
  Constant13/1 -> filtout/4(trig)
  ctrl2/1(in_arm_pack_snap) -> edge_detect/1
  edge_detect/1 -> Register1/3, Register1/1
  Register1/1 -> Logical8/2
  Logical8/1 -> Register1/2, packed_p1/3(trig), packed_p0/3(trig)
  [tvgsel_10_64] -> pipeline10/1(d)
  ctrl2/2(in_tvgsel_10_64) -> [tvgsel_10_64]
  bus_expand7/1(msb_out2) -> filtout/1(in_p0)
  bus_expand7/2(lsb_out1) -> filtout/2(in_p1)
  ctrl2/3(in_trig_adc_snaps) -> [trig_adc_snap]
  pipeline10/1(q) -> 10_to_64_new/5(tvg_sel)
  ctrl2/4(in_trig_up_snaps) -> [trig_up_snap]
  counter5/1 -> Convert2/1
  [spead_dv0] -> Logical11/1, Logical9/1, Logical/1
  Logical/1 -> [s64_v0]
  Inverter6/1 -> Logical/2
  Logical9/1 -> [s64_v1]
  Logical11/1 -> counter5/1
  [spead_eof0] -> Logical11/2
  counter6/1 -> Convert/1
  [spead_dv1] -> Logical12/1, Logical14/1, Logical13/1
  Logical12/1 -> [s64_v2]
  Inverter7/1 -> Logical12/2
  Logical14/1 -> [s64_v3]
  Logical13/1 -> counter6/1
  [spead_eof1] -> Logical13/2
  gbe_iptx2/1(in_reg) -> [s64_ip2]
  gbe_iptx3/1(in_reg) -> [s64_ip3]
  Constant2/1 -> gbe_iptx2/1(sim_1)
  Constant3/1 -> gbe_iptx3/1(sim_1)
  Convert/1 -> Inverter7/1, Logical14/2
  Convert2/1 -> Inverter6/1, Logical9/2
  gbe0/1(led_up) -> [up_gbe0]
  gbe0/2(led_rx) -> [rx_gbe0]
  gbe0/3(led_tx) -> [tx_gbe0]
  gbe0/5(tx_overflow) -> [tx_over_gbe0]
  gbe0/12(rx_overrun) -> [rxover_gbe0]
  gbe0/11(rx_bad_frame) -> [rxbad_gbe0]
  gbe0/6(rx_data) -> [rxdata_gbe0]
  gbe0/7(rx_valid) -> [rxvld_gbe0]
  gbe0/8(rx_source_ip) -> [rxip_gbe0]
  gbe0/9(rx_source_port) -> [rxport_gbe0]
  gbe0/10(rx_end_of_frame) -> [rxeof_gbe0]
  [gbe_rst] -> pipeline102/1(d)
  gbe1/1(led_up) -> [up_gbe1]
  gbe1/2(led_rx) -> [rx_gbe1]
  gbe1/3(led_tx) -> [tx_gbe1]
  gbe1/4(tx_afull) -> [tx_full_gbe1]
  gbe1/5(tx_overflow) -> [tx_over_gbe1]
  gbe1/12(rx_overrun) -> [rxover_gbe1]
  gbe1/11(rx_bad_frame) -> [rxbad_gbe1]
  gbe1/6(rx_data) -> [rxdata_gbe1]
  gbe1/7(rx_valid) -> [rxvld_gbe1]
  gbe1/8(rx_source_ip) -> [rxip_gbe1]
  gbe1/9(rx_source_port) -> [rxport_gbe1]
  gbe1/10(rx_end_of_frame) -> [rxeof_gbe1]
  gbe2/1(led_up) -> [up_gbe2]
  gbe2/2(led_rx) -> [rx_gbe2]
  gbe2/3(led_tx) -> [tx_gbe2]
  gbe2/4(tx_afull) -> [tx_full_gbe2]
  gbe2/5(tx_overflow) -> [tx_over_gbe2]
  gbe2/12(rx_overrun) -> [rxover_gbe2]
  gbe2/11(rx_bad_frame) -> [rxbad_gbe2]
  gbe2/6(rx_data) -> [rxdata_gbe2]
  gbe2/7(rx_valid) -> [rxvld_gbe2]
  gbe2/8(rx_source_ip) -> [rxip_gbe2]
  gbe2/9(rx_source_port) -> [rxport_gbe2]
  gbe2/10(rx_end_of_frame) -> [rxeof_gbe2]
  gbe3/1(led_up) -> [up_gbe3]
  gbe3/2(led_rx) -> [rx_gbe3]
  gbe3/3(led_tx) -> [tx_gbe3]
  gbe3/4(tx_afull) -> [tx_full_gbe3]
  gbe3/5(tx_overflow) -> [tx_over_gbe3]
  gbe3/12(rx_overrun) -> [rxover_gbe3]
  gbe3/11(rx_bad_frame) -> [rxbad_gbe3]
  gbe3/6(rx_data) -> [rxdata_gbe3]
  gbe3/7(rx_valid) -> [rxvld_gbe3]
  gbe3/8(rx_source_ip) -> [rxip_gbe3]
  gbe3/9(rx_source_port) -> [rxport_gbe3]
  gbe3/10(rx_end_of_frame) -> [rxeof_gbe3]
  gbe0/4(tx_afull) -> [tx_full_gbe0]
  edge_detect7/1(out) -> pipeline7/1(d)
  [sys_rst] -> edge_detect11/1(in)
  [rxdata_gbe0] -> concat0/1
  [rxdata_gbe1] -> concat0/2
  [rxdata_gbe2] -> concat0/3
  [rxdata_gbe3] -> concat0/4
  [rxeof_gbe0] -> concat1/1
  [rxeof_gbe1] -> concat1/2
  [rxeof_gbe2] -> concat1/3
  [rxeof_gbe3] -> concat1/4
  [rxvld_gbe0] -> concat3/1
  [rxvld_gbe1] -> concat3/2
  [rxvld_gbe2] -> concat3/3
  [rxvld_gbe3] -> concat3/4
  bus_expand2/4(lsb_out1) -> [unpack_adc_or1]
  control/6(in_cnt_rst) -> edge_detect2/1(in)
  concat0/1 -> unpack_and_reorder/2(din)
  concat1/1 -> unpack_and_reorder/3(eof)
  concat3/1 -> unpack_and_reorder/4(en)
  constant/1 -> unpack_and_reorder/5(transmit)
  unpack_and_reorder/4(timestamp) -> Delay11/1
  unpack_and_reorder/5(recvd) -> bus_expand17/1(bus_in)
  unpack_and_reorder/1(sync) -> Delay16/1
  edge_detect2/1(out) -> pipeline14/1(d)
  control/3(in_gbe_rst) -> pipeline19/1(d)
  control/1(in_sys_rst) -> pipeline/1(d)
  Constant14/1 -> gbe1/8(rx_overrun_ack), gbe1/7(rx_ack)
  [gbe_rst] -> pipeline104/1(d)
  Constant23/1 -> gbe2/8(rx_overrun_ack), gbe2/7(rx_ack)
  [gbe_rst] -> pipeline103/1(d)
  Constant33/1 -> gbe3/7(rx_ack), gbe3/8(rx_overrun_ack)
  [gbe_rst] -> pipeline101/1(d)
  Constant20/1 -> gbe0/8(rx_overrun_ack), gbe0/7(rx_ack)
  [gbe_cnt_rst] -> pipeline93/1(d)
  [gbe_cnt_rst] -> pipeline100/1(d)
  [gbe_cnt_rst] -> pipeline98/1(d)
  [gbe_cnt_rst] -> pipeline99/1(d)
  pipeline/1(q) -> [sys_rst]
  pipeline7/1(q) -> [clr_status]
  pipeline19/1(q) -> [gbe_rst]
  pipeline29/1(q) -> [gbe_txen]
  pipeline13/1(q) -> [tvg_adc_en]
  pipeline14/1(q) -> [cnt_rst]
  control/5(in_tvg_adc) -> pipeline13/1(d)
  edge_detect4/1(out) -> pipeline33/1(d)
  pipeline33/1(q) -> [gbe_cnt_rst]
  control/7(in_gbe_cnt_rst) -> edge_detect4/1(in)
  [s64_d0] -> pipeline5/1(d)
  [s64_ip0] -> pipeline22/1(d)
  [s64_port] -> pipeline6/1(d)
  unpack_and_reorder/2(dout) -> Delay17/1
  unpack_and_reorder/10(discarding) -> Delay19/1
  unpack_and_reorder/11(timestep_error) -> Delay29/1
  sync_gen/2(dout) -> bus_expand6/1(bus_in)
  sync_gen/3(dvalid) -> impulse_gen1/6(en), impulse_gen0/6(en)
  Slice/1 -> pipeline16/1(d)
  pipeline16/1(q) -> local_time_lsw/1(out_timestamp_lsw)
  Slice16/1 -> Convert1/1
  pipeline47/1(q) -> local_time_msw/1(out_timestamp_msw)
  Convert1/1 -> pipeline47/1(d)
  Concat2/1 -> Slice16/1, [time80_48], Slice/1
  [time80] -> Concat2/1
  Constant53/1 -> Concat2/2
  control/4(in_gbe_txen) -> pipeline29/1(d)
  control/2(in_status_clr) -> edge_detect7/1(in)
  edge_detect11/1(out) -> unpack_and_reorder/1(rst)
  [cnt_rst] -> Subsystem/1(rst)
  unpack_and_reorder/12(mcnt_relock) -> Delay30/1
  [unpack_recvd0] -> Inverter1/1
  Inverter1/1 -> Logical10/1
  Logical10/1 -> [unpack_missing0]
  [unpack_recvd1] -> Inverter2/1
  unpack_and_reorder/3(dvalid) -> Logical10/2, Logical5/2, Delay10/1
  Inverter2/1 -> Logical5/1
  Logical5/1 -> [unpack_missing1]
  pipeline61/1(q) -> [tvg_unpack_flags_en]
  control/8(in_tvg_unpack_flags_en) -> pipeline61/1(d)
  bus_expand17/1(msb_out2) -> [unpack_recvd0]
  bus_expand17/2(lsb_out1) -> [unpack_recvd1]
  Slice12/1 -> [time80]
  impulse_gen0/3(dvalid) -> [valid80]
  impulse_gen0/1(sync_out) -> [sync80]
  impulse_gen0/2(dout) -> [d80_adc0]
  impulse_gen0/4(misco) -> Slice12/1
  [tvg_adc_en] -> impulse_gen0/1(tvg_en)
  impulse_gen1/1(sync_out) -> Terminator1/1
  impulse_gen1/2(dout) -> [d80_adc1]
  impulse_gen1/3(dvalid) -> Terminator2/1
  impulse_gen1/4(misco) -> [dig_flags]
  [tvg_adc_en] -> impulse_gen1/1(tvg_en)
  impulse0/1(in_offset) -> Slice10/1
  impulse0/2(in_amplitude) -> impulse_gen0/3(impulse_amplitude)
  impulse1/1(in_offset) -> Slice11/1
  impulse1/2(in_amplitude) -> impulse_gen1/3(impulse_amplitude)
  sync_gen/1(sync) -> impulse_gen1/4(sync_in), impulse_gen0/4(sync_in)
  bus_expand6/1(msb_out2) -> impulse_gen0/5(din)
  bus_expand6/2(lsb_out1) -> impulse_gen1/5(din)
  sync_gen/5(misco) -> impulse_gen1/7(misci)
  sync_gen/4(time_out) -> impulse_gen0/7(misci)
  pipeline93/1(q) -> gbe0/9(debug_rst)
  pipeline98/1(q) -> gbe2/9(debug_rst)
  pipeline99/1(q) -> gbe3/9(debug_rst)
  pipeline100/1(q) -> gbe1/9(debug_rst)
  pipeline101/1(q) -> gbe0/1(rst)
  pipeline102/1(q) -> gbe1/1(rst)
  pipeline103/1(q) -> gbe3/1(rst)
  pipeline104/1(q) -> gbe2/1(rst)
  [s64_d2] -> pipeline30/1(d)
  [s64_ip2] -> pipeline32/1(d)
  [s64_port] -> pipeline36/1(d)
  [s64_ip1] -> pipeline40/1(d)
  [s64_port] -> pipeline41/1(d)
  [s64_d1] -> pipeline37/1(d)
  [s64_d3] -> pipeline46/1(d)
  [s64_ip3] -> pipeline48/1(d)
  [s64_port] -> pipeline49/1(d)
  [gbe_txen] -> Delay/1
  [s64_eof0] -> Delay/2
  pipeline5/1(q) -> gbe0/2(tx_data)
  pipeline22/1(q) -> gbe0/4(tx_dest_ip)
  pipeline6/1(q) -> gbe0/5(tx_dest_port)
  [gbe_txen] -> Delay28/1
  [gbe_txen] -> Delay31/1
  [gbe_txen] -> Delay32/1
  [s64_eof2] -> Delay28/2
  [s64_eof3] -> Delay32/2
  [s64_eof1] -> Delay31/2
  Logical1/1 -> gbe0/3(tx_valid)
  Logical6/1 -> gbe1/3(tx_valid)
  Logical7/1 -> gbe3/3(tx_valid)
  Logical16/1 -> gbe3/6(tx_end_of_frame)
  Logical17/1 -> gbe2/6(tx_end_of_frame)
  Logical18/1 -> gbe2/3(tx_valid)
  Logical19/1 -> gbe1/6(tx_end_of_frame)
  Delay31/1 -> Logical6/1, Logical19/1
  [s64_eof1] -> Logical19/2
  [s64_v1] -> Logical6/2
  [s64_v0] -> Logical1/2
  [s64_v2] -> Logical18/2
  [s64_eof2] -> Logical17/2
  [s64_eof3] -> Logical16/2
  [s64_v3] -> Logical7/2
  Delay32/1 -> Logical16/1, Logical7/1
  Delay28/1 -> Logical17/1, Logical18/1
  Logical3/1 -> gbe0/6(tx_end_of_frame)
  Delay/1 -> Logical1/1, Logical3/1
  [s64_eof0] -> Logical3/2
  Constant31/1 -> Concat9/2
  [unpack_timestamp] -> Concat9/1
  pipeline122/1(q) -> [tvg_pfb_flags_en]
  control/9(in_tvg_pfb_flags_en) -> pipeline122/1(d)
  unpack_and_reorder/6(flags) -> Delay18/1
  bus_expand2/1(msb_out4) -> [unpack_ndiode0]
  bus_expand2/2(out3) -> [unpack_adc_or0]
  bus_expand2/3(out2) -> [unpack_ndiode1]
  unpack_and_reorder/7(fifo_of) -> Relational3/1
  Constant21/1 -> Relational3/2
  Relational3/1 -> [unpack_fifo_of]
  Constant34/1 -> Relational4/2
  unpack_and_reorder/8(packet_of) -> Delay35/1, Relational4/1
  Relational4/1 -> [unpack_fifo_pktof]
  Constant35/1 -> Relational5/2
  unpack_and_reorder/9(spead_error) -> Delay34/1, Relational5/1
  Relational5/1 -> [unpack_spead_error]
  Constant36/1 -> Relational6/2
  [unpack_missing0] -> Concat14/1
  [unpack_missing1] -> Concat14/2
  Concat14/1 -> Relational6/1
  Relational6/1 -> [unpack_missing]
  [timestep_error] -> Logical15/1
  [sys_rst] -> Logical15/2
  Logical15/1 -> edge_detect17/1(in)
  edge_detect17/1(out) -> [sys_relock]
  [unpack_fifo_pktof] -> Concat11/5
  [unpack_spead_error] -> Concat11/7
  [unpack_discarding] -> Concat11/4
  [unpack_mcnt_relock] -> Concat11/3
  [unpack_adc_or0] -> Concat11/8
  [unpack_adc_or1] -> Concat11/9
  [unpack_fifo_of] -> Concat11/6
  [unpack_ndiode0] -> Concat11/10
  [unpack_ndiode1] -> Concat11/11
  [unpack_missing] -> Concat11/2
  [timestep_error] -> Concat11/1
  bus_expand18/1(msb_out4) -> [up_spead_error0]
  bus_expand18/2(out3) -> [up_spead_error1]
  bus_expand18/3(out2) -> [up_spead_error2]
  bus_expand18/4(lsb_out1) -> [up_spead_error3]
  [up_spead_error0] -> Subsystem/6(error0)
  [up_spead_error1] -> Subsystem/7(error1)
  [up_spead_error2] -> Subsystem/8(error2)
  [up_spead_error3] -> Subsystem/9(error3)
  bus_expand20/1(msb_out4) -> [upfifo_of0]
  bus_expand20/2(out3) -> [upfifo_of1]
  bus_expand20/3(out2) -> [upfifo_of2]
  bus_expand20/4(lsb_out1) -> [upfifo_of3]
  [up_gbe0] -> pipeline3/1(d)
  [up_gbe1] -> pipeline15/1(d)
  [up_gbe2] -> pipeline34/1(d)
  [up_gbe3] -> pipeline35/1(d)
  pipeline3/1(q) -> status/1(out_gbe0_linkup)
  pipeline15/1(q) -> status/2(out_gbe1_linkup)
  pipeline34/1(q) -> status/3(out_gbe2_linkup)
  pipeline35/1(q) -> status/4(out_gbe3_linkup)
  Subsystem/4(ctr3) -> spead_ctrs/4(out_rx_cnt3)
  Subsystem/2(ctr1) -> spead_ctrs/2(out_rx_cnt1)
  Subsystem/3(ctr2) -> spead_ctrs/3(out_rx_cnt2)
  Subsystem/5(errctr0) -> spead_ctrs/5(out_err_cnt0)
  Subsystem/1(ctr0) -> spead_ctrs/1(out_rx_cnt0)
  Subsystem/8(errctr3) -> spead_ctrs/8(out_err_cnt3)
  Subsystem/7(errctr2) -> spead_ctrs/7(out_err_cnt2)
  Subsystem/6(errctr1) -> spead_ctrs/6(out_err_cnt1)
  [up_spead_start0] -> Subsystem/2(start0)
  [up_spead_start1] -> Subsystem/3(start1)
  [up_spead_start2] -> Subsystem/4(start2)
  [up_spead_start3] -> Subsystem/5(start3)
  flag_mux0/1(timeo) -> sync_gen/1(time_in)
  [sys_relock] -> sync_gen/5(relock)
  flag_mux0/4(flagso) -> sync_gen/4(misci)
  flag_mux0/2(dvalid) -> sync_gen/2(en)
  flag_mux0/3(misco) -> sync_gen/3(din)
  [unpack_d80] -> flag_mux0/5(misci)
  [unpack_en] -> flag_mux0/3(en)
  Concat9/1 -> flag_mux0/2(timei)
  [clr_status] -> flag_mux0/1(rst)
  Concat11/1 -> flag_mux0/4(flagsi)
  tvg_flags/2(in_timestep_error) -> Concat10/1
  tvg_flags/4(in_mcnt_relock) -> Concat10/3
  tvg_flags/5(in_discarded) -> Concat10/4
  tvg_flags/6(in_pktof) -> Concat10/5
  tvg_flags/7(in_fifo_of) -> Concat10/6
  tvg_flags/8(in_spead_error) -> Concat10/7
  tvg_flags/9(in_adc_or0) -> Concat10/8
  tvg_flags/10(in_adc_or1) -> Concat10/9
  tvg_flags/11(in_ndiode0) -> Concat10/10
  tvg_flags/12(in_ndiode1) -> Concat10/11
  tvg_flags/3(in_missing) -> Concat10/2
  tvg_flags/1(in_pfb_of) -> [pfb_of]
  Concat10/1 -> flag_mux0/8(tvg_flag)
  [tvg_unpack_flags_en] -> flag_mux0/6(tvg_en)
  Constant4/1 -> flag_mux0/7(tvg_flag_default)
  Delay16/1 -> [unpack_sync]
  Delay17/1 -> [unpack_d80]
  Delay18/1 -> bus_expand2/1(bus_in)
  Delay19/1 -> [unpack_discarding]
  Delay29/1 -> [timestep_error]
  Delay30/1 -> [unpack_mcnt_relock]
  Delay34/1 -> bus_expand18/1(bus_in)
  Delay35/1 -> bus_expand20/1(bus_in)
  Slice10/1 -> impulse_gen0/2(impulse_offset)
  Slice11/1 -> impulse_gen1/2(impulse_offset)
  pipeline36/1(q) -> gbe2/5(tx_dest_port)
  pipeline32/1(q) -> gbe2/4(tx_dest_ip)
  pipeline30/1(q) -> gbe2/2(tx_data)
  pipeline41/1(q) -> gbe1/5(tx_dest_port)
  pipeline40/1(q) -> gbe1/4(tx_dest_ip)
  pipeline37/1(q) -> gbe1/2(tx_data)
  pipeline46/1(q) -> gbe3/2(tx_data)
  pipeline48/1(q) -> gbe3/4(tx_dest_ip)
  pipeline49/1(q) -> gbe3/5(tx_dest_port)
  Delay10/1 -> [unpack_en]
  Delay11/1 -> [unpack_timestamp]
  [spead_d0] -> [s64_d1], [s64_d0]
  [spead_eof0] -> [s64_eof1], [s64_eof0]
  [spead_d1] -> [s64_d2], [s64_d3]
  [spead_eof1] -> [s64_eof2], [s64_eof3]
  [cnt_rst] -> pipeline2/1(d)
  [upfifo_of0] -> pipeline18/1(d)
  [upfifo_of1] -> pipeline4/1(d)
  [upfifo_of2] -> pipeline8/1(d)
  [upfifo_of3] -> pipeline9/1(d)
  Subsystem1/1(errctr0) -> reorder_ctrs/1(out_pktof0)
  Subsystem1/2(errctr1) -> reorder_ctrs/2(out_pktof1)
  Subsystem1/3(errctr2) -> reorder_ctrs/3(out_pktof2)
  Subsystem1/4(errctr3) -> reorder_ctrs/4(out_pktof3)
  pipeline2/1(q) -> Subsystem1/1(rst)
  pipeline18/1(q) -> Subsystem1/2(error0)
  pipeline4/1(q) -> Subsystem1/3(error1)
  pipeline8/1(q) -> Subsystem1/4(error2)
  pipeline9/1(q) -> Subsystem1/5(error3)
  [unpack_missing0] -> pipeline54/1(d)
  [cnt_rst] -> Subsystem6/1(rst)
  [cnt_rst] -> pipeline11/1(d)
  [unpack_discarding] -> pipeline12/1(d)
  [timestep_error] -> pipeline26/1(d)
  [unpack_mcnt_relock] -> pipeline53/1(d)
  Subsystem5/1(errctr0) -> reorder_ctrs1/1(out_discard)
  Subsystem5/2(errctr1) -> reorder_ctrs1/2(out_timestep_error)
  Subsystem5/3(errctr2) -> reorder_ctrs1/3(out_mcnt_relock)
  edge_detect3/1 -> Subsystem6/2(error0)
  edge_detect5/1 -> Subsystem6/3(error1)
  Subsystem6/1(errctr0) -> reorder_ctrs1/4(out_recverr0)
  Subsystem6/2(errctr1) -> reorder_ctrs1/5(out_recverr1)
  [unpack_missing1] -> pipeline55/1(d)
  pipeline11/1(q) -> Subsystem5/1(rst)
  pipeline12/1(q) -> Subsystem5/2(error0)
  pipeline26/1(q) -> Subsystem5/3(error1)
  pipeline53/1(q) -> Subsystem5/4(error2)
  pipeline54/1(q) -> edge_detect3/1
  pipeline55/1(q) -> edge_detect5/1
